simulink model "doc_phasenoise"  (R2014a)
settings: Solver=VariableStepDiscrete  SolverMode=SingleTasking  StartTime=0.0  StopTime=100  RelTol=1e-3
values from neighbouring files (symbols this model uses):
  Fs = Rsym * nSamps    (= 8000000)    [commdoc_passband_mod.m]
undefined symbols (not defined in the file or in its folder): dBc, dfilt, Hz
libraries: dspsigops x5, dspsnks4 x4, dspstat3 x3, dspspect3 x2, dsparch4 x2, commrflib2 x1, dspsrcs4 x1
settings Model: Creator=The MathWorks Inc.
settings DataIOCC: SignalLoggingSaveFormat=ModelDataLogs  SaveOutput=off  SaveTime=off
settings OptimizationCC: BooleanDataType=off  InlineParams=on  ExpressionDepthLimit=2147483647  LocalBlockOutputs=off
settings DebuggingCC: AlgebraicLoopMsg=error  UnderspecifiedInitializationDetection=Classic  SingleTaskRateTransMsg=error  FcnCallInpInsideContextMsg=EnableAllAsWarning  StateNameClashWarn=warning

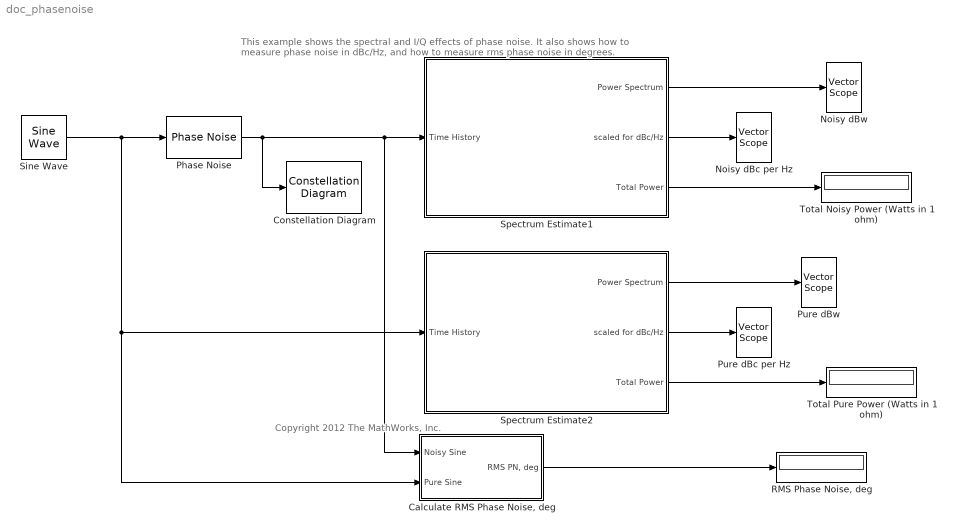
== system doc_phasenoise ==
  note: This example shows the spectral and I/Q effects of phase noise.
      | It also shows how to measure phase noise in dBc/Hz, and
      | how to measure rms phase noise in degrees.
  note: Copyright 2012 The MathWorks, Inc.
  "Calculate RMS Phase Noise, deg" : Subsystem
  Constellation Diagram : ConstellationDiagram  Tag=ScatterPlot
  Noisy dBc per Hz : dspsnks4/Vector Scope  ScopeProperties=on  Domain=Frequency  HorizSpan=1  DisplayProperties=off  AxisGrid=on  Memory=off  FrameNumber=on  AxisLegend=off  AxisZoom=off  OpenScopeAtSimStart=on  OpenScopeImmediately=off  FigPos=[422 54 363 235]  AxisProperties=off  XUnits=Hertz  XRange=[-Fs/2...Fs/2]  InheritXIncr=on  XIncr=1/8192  XLabel=Time  XLimit=Auto  XMin=-512  XMax=512  XStart=0  YUnits=dB  YLabel=dBc/Hz  LineProperties=off  XAxisParamsVer=6.9
      settings: YMin=-150  YMax=10
  Noisy dBw : dspsnks4/Vector Scope  ScopeProperties=on  Domain=Frequency  HorizSpan=1  DisplayProperties=off  AxisGrid=on  Memory=off  FrameNumber=on  AxisLegend=off  AxisZoom=off  OpenScopeAtSimStart=on  OpenScopeImmediately=off  FigPos=[17 53 386 235]  AxisProperties=off  XUnits=Hertz  XRange=[-Fs/2...Fs/2]  InheritXIncr=on  XIncr=1  XLabel=Time  XLimit=Auto  XMin=-512  XMax=512  XStart=0  YUnits=dB  YLabel=dBw  LineProperties=off  XAxisParamsVer=6.9
      settings: YMin=-100  YMax=10
  Phase Noise : commrflib2/Phase Noise  PhNs=[-60 -80]  Fo=[20 200]  Fs=8192  seed=2137
      settings: AttributesFormatString=\n
  Pure dBc per Hz : dspsnks4/Vector Scope  ScopeProperties=on  Domain=Frequency  HorizSpan=1  DisplayProperties=off  AxisGrid=on  Memory=off  FrameNumber=on  AxisLegend=off  AxisZoom=off  OpenScopeAtSimStart=on  OpenScopeImmediately=off  FigPos=[418 437 367 238]  AxisProperties=off  XUnits=Hertz  XRange=[-Fs/2...Fs/2]  InheritXIncr=on  XIncr=1  XLabel=Time  XLimit=Auto  XMin=-512  XMax=512  XStart=0  YUnits=dB  YLabel=dBc/Hz  LineProperties=off  XAxisParamsVer=6.9
      settings: YMin=-402.0216  YMax=8.0015
  Pure dBw : dspsnks4/Vector Scope  ScopeProperties=on  Domain=Frequency  HorizSpan=1  DisplayProperties=off  AxisGrid=on  Memory=off  FrameNumber=on  AxisLegend=off  AxisZoom=off  OpenScopeAtSimStart=on  OpenScopeImmediately=off  FigPos=[14 435 385 241]  AxisProperties=off  XUnits=Hertz  XRange=[-Fs/2...Fs/2]  InheritXIncr=on  XIncr=1  XLabel=Time  XLimit=Auto  XMin=-512  XMax=512  XStart=0  YUnits=dB  YLabel=dBw  LineProperties=off  XAxisParamsVer=6.9
      settings: YMin=-400.2607  YMax=9.7625
  "RMS Phase Noise, deg" : Display
  Sine Wave : dspsrcs4/Sine Wave  Amplitude=1  Frequency=128  Phase=pi/8  SampleMode=Discrete  OutComplex=Complex  CompMethod=Trigonometric fcn  TableSize=Speed  SampleTime=1/8192  SamplesPerFrame=1024  ResetState=Restart at time zero  dataType=double  wordLen=16  udDataType=sfix(16)  fracBitsMode=Best precision  numFracBits=15  OutDataTypeStr=double  LastOutDataTypeStr=double
  Spectrum Estimate1 : Subsystem  mask{Frame=1024, Navg=400}
      mask prompts: Frame "Frame Size"
      mask Display:
      | disp('Power Spectrum \n Estimate')
      | port_label('input',1,'y(t)');
      | port_label('output',1,'Power Spectrum')
      | port_label('output',2,'Scaled for dBc/Hz')
      | port_label('output',3','Total Power');
  Spectrum Estimate2 : Subsystem  mask{Frame=1024, Navg=400}
      mask prompts: Frame "Frame Size"
      mask Display:
      | disp('Power Spectrum \n Estimate')
      | port_label('input',1,'y(t)');
      | port_label('output',1,'Power Spectrum')
      | port_label('output',2,'Scaled for dBc/Hz')
      | port_label('output',3','Total Power');
  Total Noisy Power (Watts in 1 ohm) : Display
  Total Pure Power (Watts in 1 ohm) : Display
  wires:
  Sine Wave/1 -> Phase Noise/1, Spectrum Estimate2/1(Time History), "Calculate RMS Phase Noise, deg"/2(Pure Sine)
  Phase Noise/1 -> Spectrum Estimate1/1(Time History), "Calculate RMS Phase Noise, deg"/1(Noisy Sine), Constellation Diagram/1
  Spectrum Estimate1/1(Power Spectrum) -> Noisy dBw/1
  Spectrum Estimate1/2(scaled for dBc/Hz) -> Noisy dBc per Hz/1
  Spectrum Estimate1/3(Total Power) -> Total Noisy Power (Watts in 1 ohm)/1
  Spectrum Estimate2/1(Power Spectrum) -> Pure dBw/1
  Spectrum Estimate2/2(scaled for dBc/Hz) -> Pure dBc per Hz/1
  Spectrum Estimate2/3(Total Power) -> Total Pure Power (Watts in 1 ohm)/1
  "Calculate RMS Phase Noise, deg"/1("RMS PN, deg") -> "RMS Phase Noise, deg"/1

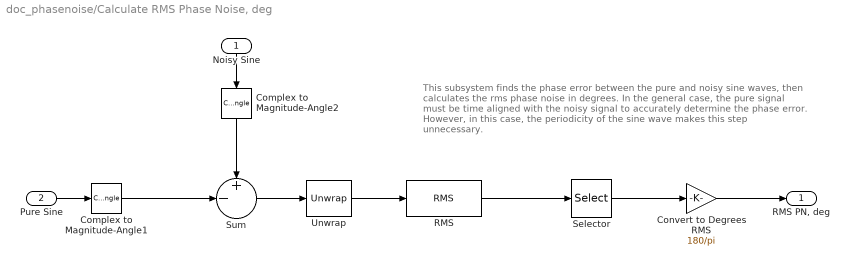
== system doc_phasenoise/Calculate RMS Phase Noise, deg ==
  note: This subsystem finds the phase error between the pure and noisy sine waves,
      | then calculates the rms phase noise in degrees.  In the general case, the
      | pure signal must be time aligned with the noisy signal to accurately determine
      | the phase error.  However, in this case, the periodicity of the sine wave makes
      | this step unnecessary.
  Noisy Sine : Inport
  Pure Sine : Inport  Port=2
  Complex to Magnitude-Angle1 : ComplexToMagnitudeAngle  Output=Angle
  Complex to Magnitude-Angle2 : ComplexToMagnitudeAngle  Output=Angle
  Convert to Degrees RMS : Gain  Gain=180/pi
  RMS : dspstat3/RMS  run=on  reset_popup=None  InputProcessing=Columns as channels (frame based)  directionMode=Each column  dimension=1  treatSBRowAsCol=on
  Selector : Selector  NumberOfDimensions=2  InputPortWidth=3  IndexOptions=Index vector (dialog),Index vector (dialog)  Indices=1024,1  OutputSizes=1,1
  Sum : Sum  Inputs=+-|
  Unwrap : dspsigops/Unwrap  tol=pi  InputProcessing=Columns as channels (frame based)  running=off
  "RMS PN, deg" : Outport
  wires:
  Sum/1 -> Unwrap/1
  RMS/1 -> Selector/1
  Selector/1 -> Convert to Degrees RMS/1
  Complex to Magnitude-Angle1/1 -> Sum/2
  Complex to Magnitude-Angle2/1 -> Sum/1
  Noisy Sine/1 -> Complex to Magnitude-Angle2/1
  Pure Sine/1 -> Complex to Magnitude-Angle1/1
  Convert to Degrees RMS/1 -> "RMS PN, deg"/1
  Unwrap/1 -> RMS/1

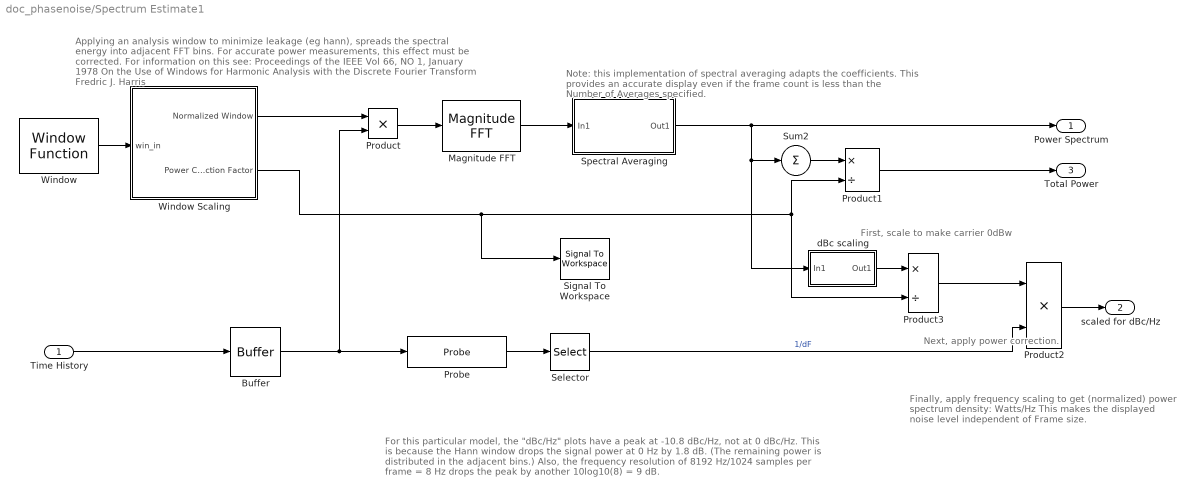
== system doc_phasenoise/Spectrum Estimate1 ==
  note: For this particular model, the "dBc/Hz" plots have a peak at -10.8 dBc/Hz, not
      | at 0 dBc/Hz.  This is because the Hann window drops the signal power at 0 Hz by 1.8 dB.
      | (The remaining power is distributed in the adjacent bins.)  Also, the frequency resolution
      | of 8192 Hz/1024 samples per frame = 8 Hz drops the peak by another 10log10(8) = 9 dB.
  note: Applying an analysis window to minimize leakage (eg hann),
      | spreads the spectral energy into adjacent FFT bins.
      | For accurate power measurements, this effect must be corrected.
      | For information on this see:
      | Proceedings of the IEEE Vol 66, NO 1, January 1978
      | On the Use of Windows for Harmonic Analysis with the Discrete Fourier Transform
      | Fredric J. Harris
  note: Next, apply power correction.
  note: First, scale to make carrier 0dBw
  note: Note: this implementation of spectral averaging adapts the coefficients.
      | This provides an accurate display even if the frame
      | count is less than the Number of Averages specified.
  note: Finally, apply frequency scaling
      | to get (normalized) power spectrum density: Watts/Hz
      | This makes the displayed noise level independent
      | of Frame size.
  Time History : Inport
  Buffer : Buffer  N=Frame  TreatMby1Signals=One channel
  Magnitude FFT : dspspect3/Magnitude FFT  mag_or_magsq=Magnitude squared  FFTImplementation=Auto  fftLenInherit=on  fftsize=fftsize  WrapInput=on
  Probe : Probe  ProbeWidth=off  ProbeComplexSignal=off  ProbeWidthDataType=single  ProbeSampleTimeDataType=single
  Product : Product  RndMeth=Zero
  Product1 : Product  Inputs=*/  RndMeth=Zero
  Product2 : Product  Inputs=**  RndMeth=Zero
  Product3 : Product  Inputs=*/  RndMeth=Zero
  Selector : Selector  InputPortWidth=2  Indices=[1]
  Signal To Workspace : SignalToWorkspace  VariableName=pwr_corr
      settings: CopyFcn=dspblkcopystw(gcbh);
  Spectral Averaging : Subsystem  mask{Navg=Navg}
      mask Display: disp('Spectral Averaging')
  Sum2 : Sum  Inputs=+
  Window : dspsigops/Window Function  winmode=Generate window  wintype=Hann  sampmode=Discrete  samptime=inf  N=Frame  Rs=60  beta=1  winsamp=Periodic  UserWindow=hamming  OptParams=off  UserParams={1.0}  RowConvenienceOn=on  dataType=double  isSigned=on  wordLen=16  udDataType=sfix(16)  fracBitsMode=Best precision  numFracBits=15  roundingMode=Floor  overflowMode=off  numSidelobes=4  sidelobeLevel=-30
      settings: additionalParams=on
  Window Scaling : Subsystem
  dBc scaling : Subsystem
  Power Spectrum : Outport
  scaled for dBc/Hz : Outport  Port=2
  Total Power : Outport  Port=3
  wires:
  Product3/1 -> Product2/1
  dBc scaling/1(Out1) -> Product3/1
  Window/1 -> Window Scaling/1(win_in)
  Window Scaling/1(Normalized Window) -> Product/1
  Buffer/1 -> Product/2, Probe/1
  Selector/1 -> Product2/2  "1/dF"
  Product2/1 -> scaled for dBc/Hz/1
  Probe/1 -> Selector/1
  Time History/1 -> Buffer/1
  Spectral Averaging/1(Out1) -> dBc scaling/1(In1), Sum2/1, Power Spectrum/1
  Product1/1 -> Total Power/1
  Sum2/1 -> Product1/1
  Window Scaling/2(Power Correction Factor) -> Product1/2, Product3/2, Signal To Workspace/1
  Magnitude FFT/1 -> Spectral Averaging/1(In1)
  Product/1 -> Magnitude FFT/1

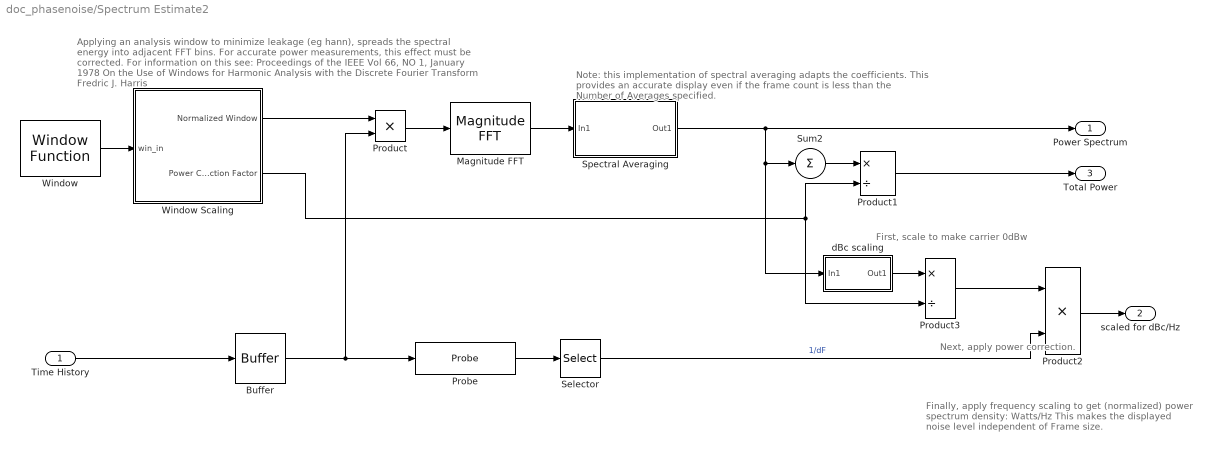
== system doc_phasenoise/Spectrum Estimate2 ==
  note: Finally, apply frequency scaling
      | to get (normalized) power spectrum density: Watts/Hz
      | This makes the displayed noise level independent
      | of Frame size.
  note: Note: this implementation of spectral averaging adapts the coefficients.
      | This provides an accurate display even if the frame
      | count is less than the Number of Averages specified.
  note: First, scale to make carrier 0dBw
  note: Next, apply power correction.
  note: Applying an analysis window to minimize leakage (eg hann),
      | spreads the spectral energy into adjacent FFT bins.
      | For accurate power measurements, this effect must be corrected.
      | For information on this see:
      | Proceedings of the IEEE Vol 66, NO 1, January 1978
      | On the Use of Windows for Harmonic Analysis with the Discrete Fourier Transform
      | Fredric J. Harris
  Time History : Inport
  Buffer : Buffer  N=Frame  TreatMby1Signals=One channel
  Magnitude FFT : dspspect3/Magnitude FFT  mag_or_magsq=Magnitude squared  FFTImplementation=Auto  fftLenInherit=on  fftsize=fftsize  WrapInput=on
  Probe : Probe  ProbeWidth=off  ProbeComplexSignal=off  ProbeWidthDataType=single  ProbeSampleTimeDataType=single
  Product : Product  RndMeth=Zero
  Product1 : Product  Inputs=*/  RndMeth=Zero
  Product2 : Product  Inputs=**  RndMeth=Zero
  Product3 : Product  Inputs=*/  RndMeth=Zero
  Selector : Selector  InputPortWidth=2  Indices=[1]
  Spectral Averaging : Subsystem  mask{Navg=Navg}
      mask Display: disp('Spectral Averaging')
  Sum2 : Sum  Inputs=+
  Window : dspsigops/Window Function  winmode=Generate window  wintype=Hann  sampmode=Discrete  samptime=inf  N=Frame  Rs=60  beta=1  winsamp=Periodic  UserWindow=hamming  OptParams=off  UserParams={1.0}  RowConvenienceOn=on  dataType=double  isSigned=on  wordLen=16  udDataType=sfix(16)  fracBitsMode=Best precision  numFracBits=15  roundingMode=Floor  overflowMode=off  numSidelobes=4  sidelobeLevel=-30
      settings: additionalParams=on
  Window Scaling : Subsystem
  dBc scaling : Subsystem
  Power Spectrum : Outport
  scaled for dBc/Hz : Outport  Port=2
  Total Power : Outport  Port=3
  wires:
  Product/1 -> Magnitude FFT/1
  Magnitude FFT/1 -> Spectral Averaging/1(In1)
  Window Scaling/2(Power Correction Factor) -> Product3/2, Product1/2
  Sum2/1 -> Product1/1
  Product1/1 -> Total Power/1
  Spectral Averaging/1(Out1) -> Power Spectrum/1, Sum2/1, dBc scaling/1(In1)
  Time History/1 -> Buffer/1
  Probe/1 -> Selector/1
  Product2/1 -> scaled for dBc/Hz/1
  Selector/1 -> Product2/2  "1/dF"
  Buffer/1 -> Probe/1, Product/2
  Window Scaling/1(Normalized Window) -> Product/1
  Window/1 -> Window Scaling/1(win_in)
  dBc scaling/1(Out1) -> Product3/1
  Product3/1 -> Product2/1

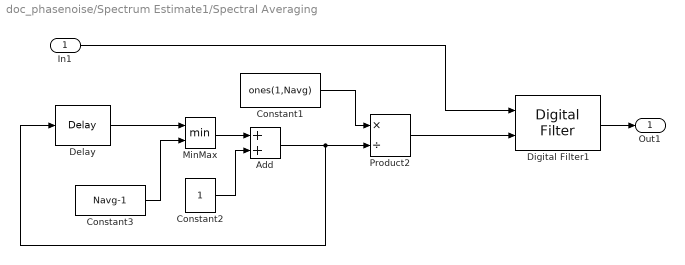
== system doc_phasenoise/Spectrum Estimate1/Spectral Averaging ==
  In1 : Inport
  Add : Sum
  Constant1 : Constant  Value=ones(1,Navg)  OutDataTypeStr=double
  Constant2 : Constant  OutDataTypeStr=double
  Constant3 : Constant  Value=Navg-1  OutDataTypeStr=double
  Delay : dspsigops/Delay  InputProcessing=Inherited (this choice will be removed - see release notes)  dly_unit=Samples  delay=1  ic_detail=off  dif_ic_for_ch=off  dif_ic_for_dly=off  ic=0  reset_popup=None
  Digital Filter1 : dsparch4/Digital Filter  TypePopup=FIR (all zeros)  IIRFiltStruct=Direct form II transposed  AllPoleFiltStruct=Direct form  FIRFiltStruct=Direct form  CoeffSource=Input port(s)  NumCoeffs=[1 2]  DenCoeffs=[1 0.1]  BiQuadCoeffs=[1 0.3 0.4 1 0.1 0.2]  LatticeCoeffs=[0.2 0.4]  denIgnore=on  FiltPerSampPopup=One filter per frame  IC=0  ICnum=0  ICden=0  roundingMode=Floor  overflowMode=off  ScaleValues=1  scaleValueFracLength=14  stageInFracLength=15  stageOutFracLength=15  FilterSource=Input port(s)  dfiltObjectName=dfilt.dffir([1 2 1])
  MinMax : MinMax  Inputs=2
  Product2 : Product  Inputs=*/  RndMeth=Zero
  Out1 : Outport
  wires:
  Constant1/1 -> Product2/1
  Digital Filter1/1 -> Out1/1
  In1/1 -> Digital Filter1/1
  Constant3/1 -> MinMax/2
  MinMax/1 -> Add/1
  Delay/1 -> MinMax/1
  Product2/1 -> Digital Filter1/2
  Constant2/1 -> Add/2
  Add/1 -> Product2/2, Delay/1

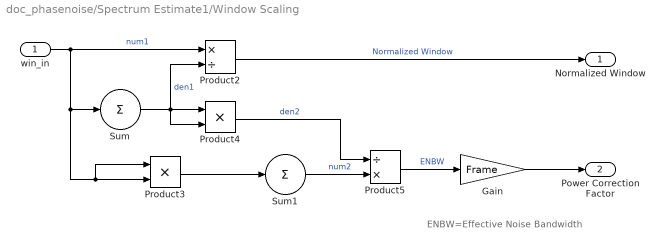
== system doc_phasenoise/Spectrum Estimate1/Window Scaling ==
  note: ENBW=Effective Noise Bandwidth
  win_in : Inport
  Gain : Gain  Gain=Frame
  Product2 : Product  Inputs=*/  RndMeth=Zero
  Product3 : Product  RndMeth=Zero
  Product4 : Product  RndMeth=Zero
  Product5 : Product  Inputs=/*  RndMeth=Zero
  Sum : Sum  Inputs=+
  Sum1 : Sum  Inputs=+
  Normalized Window : Outport
  Power Correction Factor : Outport  Port=2
  wires:
  Gain/1 -> Power Correction Factor/1
  Sum/1 -> Product2/2, Product4/2, Product4/1  "den1"
  win_in/1 -> Product2/1, Product3/2, Product3/1, Sum/1  "num1"
  Product5/1 -> Gain/1  "ENBW"
  Sum1/1 -> Product5/2  "num2"
  Product4/1 -> Product5/1  "den2"
  Product3/1 -> Sum1/1
  Product2/1 -> Normalized Window/1  "Normalized Window"

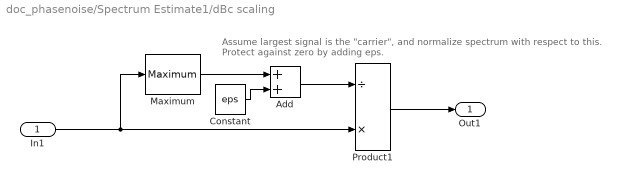
== system doc_phasenoise/Spectrum Estimate1/dBc scaling ==
  note: Assume largest signal is the "carrier", and normalize spectrum with respect to this.
      | Protect against zero by adding eps.
  In1 : Inport
  Add : Sum
  Constant : Constant  Value=eps
  Maximum : dspstat3/Maximum  fcn=Value  reset=None  InputProcessing=Columns as channels (frame based)  indexBase=One  operateOver=Each column  Dimension=1  colComp=off  operation=maximum  roiEnable=off  roiType=Rectangles  roiPortion=Entire ROI  roiOutput=Individual statistics for each ROI  roiFlag=off  accumDataTypeStr=Inherit: Same as product output  accumLastDataTypeStr=Inherit: Same as product output  roundingMode=Floor  overflowMode=off
  Product1 : Product  Inputs=/*  RndMeth=Zero
  Out1 : Outport
  wires:
  Constant/1 -> Add/2
  Maximum/1 -> Add/1
  Add/1 -> Product1/1
  Product1/1 -> Out1/1
  In1/1 -> Product1/2, Maximum/1

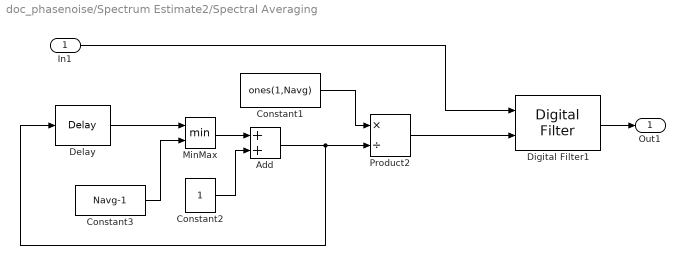
== system doc_phasenoise/Spectrum Estimate2/Spectral Averaging ==
  In1 : Inport
  Add : Sum
  Constant1 : Constant  Value=ones(1,Navg)  OutDataTypeStr=double
  Constant2 : Constant  OutDataTypeStr=double
  Constant3 : Constant  Value=Navg-1  OutDataTypeStr=double
  Delay : dspsigops/Delay  InputProcessing=Inherited (this choice will be removed - see release notes)  dly_unit=Samples  delay=1  ic_detail=off  dif_ic_for_ch=off  dif_ic_for_dly=off  ic=0  reset_popup=None
  Digital Filter1 : dsparch4/Digital Filter  TypePopup=FIR (all zeros)  IIRFiltStruct=Direct form II transposed  AllPoleFiltStruct=Direct form  FIRFiltStruct=Direct form  CoeffSource=Input port(s)  NumCoeffs=[1 2]  DenCoeffs=[1 0.1]  BiQuadCoeffs=[1 0.3 0.4 1 0.1 0.2]  LatticeCoeffs=[0.2 0.4]  denIgnore=on  FiltPerSampPopup=One filter per frame  IC=0  ICnum=0  ICden=0  roundingMode=Floor  overflowMode=off  ScaleValues=1  scaleValueFracLength=14  stageInFracLength=15  stageOutFracLength=15  FilterSource=Input port(s)  dfiltObjectName=dfilt.dffir([1 2 1])
  MinMax : MinMax  Inputs=2
  Product2 : Product  Inputs=*/  RndMeth=Zero
  Out1 : Outport
  wires:
  Add/1 -> Delay/1, Product2/2
  Constant2/1 -> Add/2
  Product2/1 -> Digital Filter1/2
  Delay/1 -> MinMax/1
  MinMax/1 -> Add/1
  Constant3/1 -> MinMax/2
  In1/1 -> Digital Filter1/1
  Digital Filter1/1 -> Out1/1
  Constant1/1 -> Product2/1

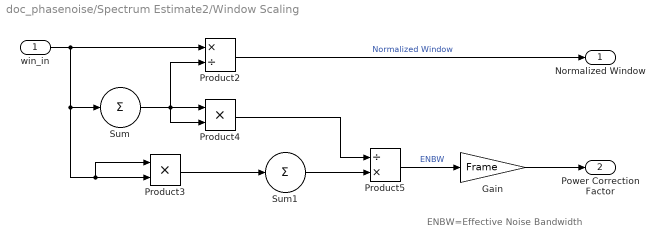
== system doc_phasenoise/Spectrum Estimate2/Window Scaling ==
  note: ENBW=Effective Noise Bandwidth
  win_in : Inport
  Gain : Gain  Gain=Frame
  Product2 : Product  Inputs=*/  RndMeth=Zero
  Product3 : Product  RndMeth=Zero
  Product4 : Product  RndMeth=Zero
  Product5 : Product  Inputs=/*  RndMeth=Zero
  Sum : Sum  Inputs=+
  Sum1 : Sum  Inputs=+
  Normalized Window : Outport
  Power Correction Factor : Outport  Port=2
  wires:
  Product2/1 -> Normalized Window/1  "Normalized Window"
  Product3/1 -> Sum1/1
  Product4/1 -> Product5/1
  Sum1/1 -> Product5/2
  Product5/1 -> Gain/1  "ENBW"
  win_in/1 -> Sum/1, Product3/1, Product3/2, Product2/1
  Sum/1 -> Product4/1, Product4/2, Product2/2
  Gain/1 -> Power Correction Factor/1

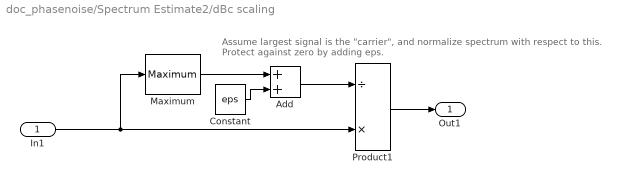
== system doc_phasenoise/Spectrum Estimate2/dBc scaling ==
  note: Assume largest signal is the "carrier", and normalize spectrum with respect to this.
      | Protect against zero by adding eps.
  In1 : Inport
  Add : Sum
  Constant : Constant  Value=eps
  Maximum : dspstat3/Maximum  fcn=Value  reset=None  InputProcessing=Columns as channels (frame based)  indexBase=One  operateOver=Each column  Dimension=1  colComp=off  operation=maximum  roiEnable=off  roiType=Rectangles  roiPortion=Entire ROI  roiOutput=Individual statistics for each ROI  roiFlag=off  accumDataTypeStr=Inherit: Same as product output  accumLastDataTypeStr=Inherit: Same as product output  roundingMode=Floor  overflowMode=off
  Product1 : Product  Inputs=/*  RndMeth=Zero
  Out1 : Outport
  wires:
  In1/1 -> Maximum/1, Product1/2
  Product1/1 -> Out1/1
  Add/1 -> Product1/1
  Maximum/1 -> Add/1
  Constant/1 -> Add/2
